simulink model "mras_square_error"  (R2019b)
settings: Solver=VariableStepAuto  StartTime=0.0  StopTime=100  RelTol=1e-3
values from neighbouring files (symbols this model uses):
  Am = [1 7 12]    [Second_order_system.m]
  b = 7    [Second_order_system.m]
  Bm = 12    [Second_order_system.m]
  gamma = 1.2    [Second_order_system.m]
settings Model: Creator=Mustafa Sezer  LastModifiedBy=Mustafa Sezer

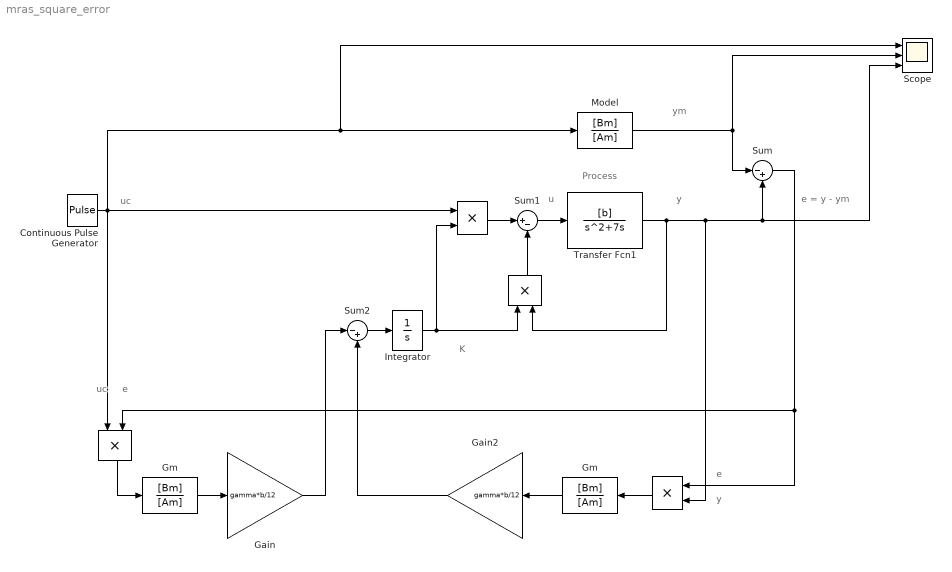
== system mras_square_error ==
  note: uc
  note: y
  note: u
  note: ym
  note: e = y - ym
  note: K
  note: Process
  note: e
  note: uc
  note: e
  note: y
  " " : Product
  " " : Product
  " " : Product
  "     " : Product
  Continuous Pulse Generator : DiscretePulseGenerator  PulseType=Time based  Period=20  PulseWidth=50
  Gain : Gain  Gain=gamma*b/12
  Gain2 : Gain  Gain=gamma*b/12
  "Gm " : TransferFcn  Numerator=[Bm]  Denominator=[Am]
  "Gm  " : TransferFcn  Numerator=[Bm]  Denominator=[Am]
  Integrator : Integrator
  Model : TransferFcn  Numerator=[Bm]  Denominator=[Am]
  Scope : Scope  NumInputPorts=3
  Sum : Sum  Inputs=|-+
  Sum1 : Sum  Inputs=|+-
  Sum2 : Sum  Inputs=|-+
  Transfer Fcn1 : TransferFcn  Numerator=[b]  Denominator=[1 7 0]
  wires:
  " "/1 -> "Gm  "/1
  Transfer Fcn1/1 -> " "/2, Sum/2, Scope/3, " "/2
  Sum1/1 -> Transfer Fcn1/1
  Model/1 -> Sum/1, Scope/2
  "     "/1 -> Sum1/1
  Continuous Pulse Generator/1 -> "     "/1, Scope/1, Model/1, " "/1
  "Gm "/1 -> Gain2/1
  " "/1 -> Sum1/2
  Gain2/1 -> Sum2/2
  Sum/1 -> " "/1, " "/2
  "Gm  "/1 -> Gain/1
  Sum2/1 -> Integrator/1
  Integrator/1 -> " "/1, "     "/2
  Gain/1 -> Sum2/1
  " "/1 -> "Gm "/1
